simulink model "realimentacao_estados"  (R2022b)
settings: Solver=VariableStepAuto  StartTime=0.0  StopTime=30  RelTol=1e-3
values from neighbouring files (symbols this model uses):
  Cd = ss_d.C    [espacoDiscreto.m]
  Dd = ss_d.D    [espacoDiscreto.m]
  disturbio = 0.24    [espacoDiscreto.m]
  F = ss_d.A    [espacoDiscreto.m]
  H = ss_d.B    [espacoDiscreto.m]
  K_ganhos = place(F,H,[0.8354 + 0.1173i,0.8354 - 0.1173i])    [espacoDiscreto.m]
  Ki = -K_ganhos_2(3)    [espacoDiscreto.m]
  R = 1.18    [espacoDiscreto.m]
  T0 = 0.203    [espacoDiscreto.m]
settings Model: Creator=coveiro  LastModifiedBy=gusta

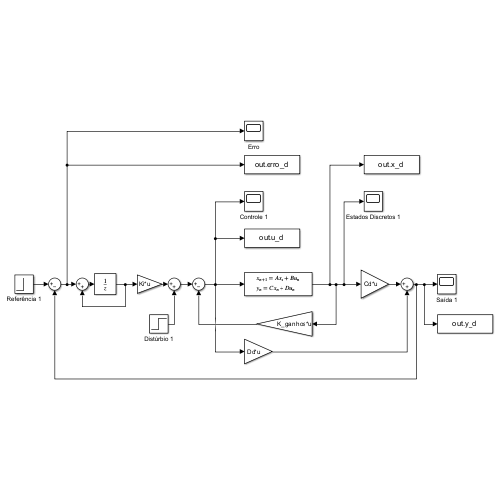
[thumbnail: Simulink's stored preview of the top-level diagram]
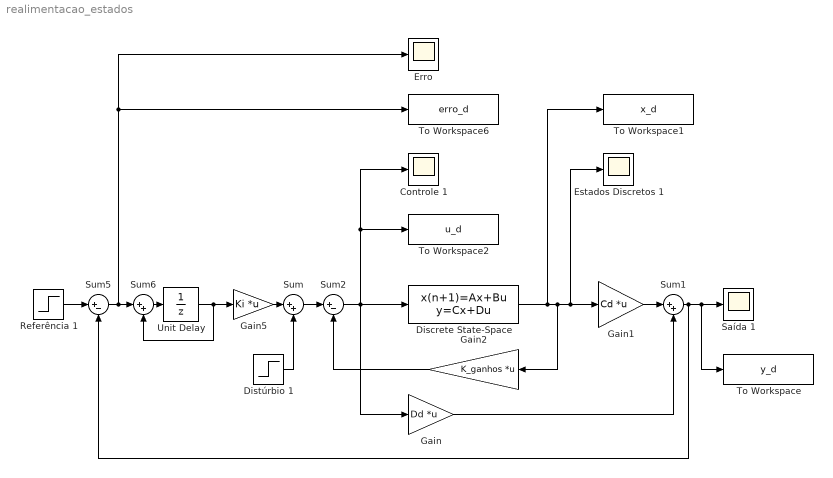
== system realimentacao_estados ==
  Controle 1 : Scope
  Discrete State-Space : DiscreteStateSpace  A=F  B=H  C=[1 0; 0 1]  D=[0;0]  SampleTime=T0
  Distúrbio 1 : Step  Time=15  After=disturbio  SampleTime=0
  Erro : Scope
  Estados Discretos 1 : Scope
  Gain : Gain  Gain=Dd  Multiplication=Matrix(K*u)
  Gain1 : Gain  Gain=Cd  Multiplication=Matrix(K*u)
  Gain2 : Gain  Gain=K_ganhos  Multiplication=Matrix(K*u)
  Gain5 : Gain  Gain=Ki  Multiplication=Matrix(K*u)
  Referência 1 : Step  Time=0  After=R  SampleTime=0
  Saída 1 : Scope
  Sum : Sum  Inputs=|++
  Sum1 : Sum  Inputs=|++
  Sum2 : Sum  Inputs=|+-
  Sum5 : Sum  Inputs=|+-
  Sum6 : Sum  Inputs=|++
  To Workspace : ToWorkspace  VariableName=y_d  SaveFormat=Timeseries  SampleTime=-1
  To Workspace1 : ToWorkspace  VariableName=x_d  SaveFormat=Timeseries  SampleTime=-1
  To Workspace2 : ToWorkspace  VariableName=u_d  SaveFormat=Timeseries  SampleTime=-1
  To Workspace6 : ToWorkspace  VariableName=erro_d  SaveFormat=Timeseries  SampleTime=-1
  Unit Delay : UnitDelay  SampleTime=-1  HasFrameUpgradeWarning=on
  wires:
  Discrete State-Space/1 -> To Workspace1/1, Gain2/1, Estados Discretos 1/1, Gain1/1
  Gain/1 -> Sum1/2
  Gain1/1 -> Sum1/1
  Sum1/1 -> To Workspace/1, Saída 1/1, Sum5/2
  Sum/1 -> Sum2/1
  Sum2/1 -> Controle 1/1, To Workspace2/1, Gain/1, Discrete State-Space/1
  Distúrbio 1/1 -> Sum/2
  Gain2/1 -> Sum2/2
  Referência 1/1 -> Sum5/1
  Sum5/1 -> To Workspace6/1, Erro/1, Sum6/1
  Unit Delay/1 -> Gain5/1, Sum6/2
  Gain5/1 -> Sum/1
  Sum6/1 -> Unit Delay/1
